simulink model "sim_model"  (R2015b)
settings: Solver=FixedStepDiscrete  SolverMode=SingleTasking  StartTime=0.0  StopTime=sim_len  FixedStep=1  RelTol=1e-3
undefined symbols (not defined in the file): A, B, C, ir_matrix, modulator_reg_1_address, modulator_reg_1_default, modulator_reg_1_num_bits, N_sub
libraries: xbsIndex_r4 x3875
(part 2 of 193)

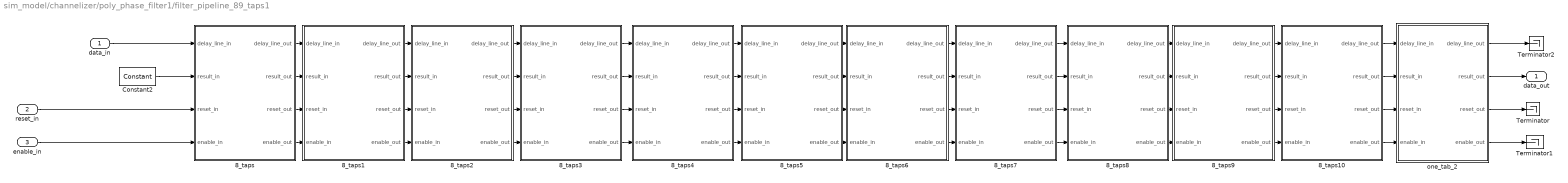
== system sim_model/channelizer/poly_phase_filter1/filter_pipeline_89_taps1 ==
  data_in : Inport
  reset_in : Inport  Port=2
  enable_in : Inport  Port=3
  8_taps : Subsystem  mask{impulse_response_matrix=impulse_response_matrix(0*8+(1:8),:), N_sub=N_sub}
      mask prompts: impulse_response_matrix "Impulse Response Matrix (N_sub x 8)"
  8_taps1 : Subsystem  mask{impulse_response_matrix=impulse_response_matrix(1*8+(1:8),:), N_sub=N_sub}
      mask prompts: impulse_response_matrix "Impulse Response Matrix (N_sub x 8)"
  8_taps10 : Subsystem  mask{impulse_response_matrix=impulse_response_matrix(10*8+(1:8),:), N_sub=N_sub}
      mask prompts: impulse_response_matrix "Impulse Response Matrix (N_sub x 8)"
  8_taps2 : Subsystem  mask{impulse_response_matrix=impulse_response_matrix(2*8+(1:8),:), N_sub=N_sub}
      mask prompts: impulse_response_matrix "Impulse Response Matrix (N_sub x 8)"
  8_taps3 : Subsystem  mask{impulse_response_matrix=impulse_response_matrix(3*8+(1:8),:), N_sub=N_sub}
      mask prompts: impulse_response_matrix "Impulse Response Matrix (N_sub x 8)"
  8_taps4 : Subsystem  mask{impulse_response_matrix=impulse_response_matrix(4*8+(1:8),:), N_sub=N_sub}
      mask prompts: impulse_response_matrix "Impulse Response Matrix (N_sub x 8)"
  8_taps5 : Subsystem  mask{impulse_response_matrix=impulse_response_matrix(5*8+(1:8),:), N_sub=N_sub}
      mask prompts: impulse_response_matrix "Impulse Response Matrix (N_sub x 8)"
  8_taps6 : Subsystem  mask{impulse_response_matrix=impulse_response_matrix(6*8+(1:8),:), N_sub=N_sub}
      mask prompts: impulse_response_matrix "Impulse Response Matrix (N_sub x 8)"
  8_taps7 : Subsystem  mask{impulse_response_matrix=impulse_response_matrix(7*8+(1:8),:), N_sub=N_sub}
      mask prompts: impulse_response_matrix "Impulse Response Matrix (N_sub x 8)"
  8_taps8 : Subsystem  mask{impulse_response_matrix=impulse_response_matrix(8*8+(1:8),:), N_sub=N_sub}
      mask prompts: impulse_response_matrix "Impulse Response Matrix (N_sub x 8)"
  8_taps9 : Subsystem  mask{impulse_response_matrix=impulse_response_matrix(9*8+(1:8),:), N_sub=N_sub}
      mask prompts: impulse_response_matrix "Impulse Response Matrix (N_sub x 8)"
  Constant2 : xbsIndex_r4/Constant  const=0  gui_display_data_type=Fixed-point  arith_type=Signed (2's comp)  n_bits=32  bin_pt=0  preci_type=Single  exp_width=8  frac_width=24  explicit_period=on  period=1  equ=P=C  opselect=C  inp2=PCIN>>17  opr=+  inp1=P  carry=CIN  dbl_ovrd=off  block_type=constant
  Terminator : Terminator
  Terminator1 : Terminator
  Terminator2 : Terminator
  one_tab_2 : Subsystem  mask{impulse_response_matrix=impulse_response_matrix(89,:), N_sub=N_sub}
      mask prompts: impulse_response_matrix "Tab IR"
  data_out : Outport
  wires:
  data_in/1 -> 8_taps/1(delay_line_in)
  reset_in/1 -> 8_taps/3(reset_in)
  enable_in/1 -> 8_taps/4(enable_in)
  Constant2/1 -> 8_taps/2(result_in)
  one_tab_2/4(enable_out) -> Terminator1/1
  one_tab_2/1(delay_line_out) -> Terminator2/1
  one_tab_2/2(result_out) -> data_out/1
  one_tab_2/3(reset_out) -> Terminator/1
  8_taps/1(delay_line_out) -> 8_taps1/1(delay_line_in)
  8_taps/2(result_out) -> 8_taps1/2(result_in)
  8_taps/3(reset_out) -> 8_taps1/3(reset_in)
  8_taps/4(enable_out) -> 8_taps1/4(enable_in)
  8_taps10/1(delay_line_out) -> one_tab_2/1(delay_line_in)
  8_taps10/2(result_out) -> one_tab_2/2(result_in)
  8_taps2/3(reset_out) -> 8_taps3/3(reset_in)
  8_taps2/4(enable_out) -> 8_taps3/4(enable_in)
  8_taps1/1(delay_line_out) -> 8_taps2/1(delay_line_in)
  8_taps1/2(result_out) -> 8_taps2/2(result_in)
  8_taps1/3(reset_out) -> 8_taps2/3(reset_in)
  8_taps1/4(enable_out) -> 8_taps2/4(enable_in)
  8_taps4/2(result_out) -> 8_taps5/2(result_in)
  8_taps4/3(reset_out) -> 8_taps5/3(reset_in)
  8_taps4/4(enable_out) -> 8_taps5/4(enable_in)
  8_taps6/3(reset_out) -> 8_taps7/3(reset_in)
  8_taps6/4(enable_out) -> 8_taps7/4(enable_in)
  8_taps5/2(result_out) -> 8_taps6/2(result_in)
  8_taps5/3(reset_out) -> 8_taps6/3(reset_in)
  8_taps5/4(enable_out) -> 8_taps6/4(enable_in)
  8_taps3/1(delay_line_out) -> 8_taps4/1(delay_line_in)
  8_taps3/2(result_out) -> 8_taps4/2(result_in)
  8_taps3/3(reset_out) -> 8_taps4/3(reset_in)
  8_taps3/4(enable_out) -> 8_taps4/4(enable_in)
  8_taps8/2(result_out) -> 8_taps9/2(result_in)
  8_taps8/3(reset_out) -> 8_taps9/3(reset_in)
  8_taps8/4(enable_out) -> 8_taps9/4(enable_in)
  8_taps9/2(result_out) -> 8_taps10/2(result_in)
  8_taps9/3(reset_out) -> 8_taps10/3(reset_in)
  8_taps9/4(enable_out) -> 8_taps10/4(enable_in)
  8_taps7/1(delay_line_out) -> 8_taps8/1(delay_line_in)
  8_taps7/2(result_out) -> 8_taps8/2(result_in)
  8_taps7/3(reset_out) -> 8_taps8/3(reset_in)
  8_taps7/4(enable_out) -> 8_taps8/4(enable_in)
  8_taps9/1(delay_line_out) -> 8_taps10/1(delay_line_in)
  8_taps10/3(reset_out) -> one_tab_2/3(reset_in)
  8_taps10/4(enable_out) -> one_tab_2/4(enable_in)
  8_taps8/1(delay_line_out) -> 8_taps9/1(delay_line_in)
  8_taps6/1(delay_line_out) -> 8_taps7/1(delay_line_in)
  8_taps6/2(result_out) -> 8_taps7/2(result_in)
  8_taps5/1(delay_line_out) -> 8_taps6/1(delay_line_in)
  8_taps4/1(delay_line_out) -> 8_taps5/1(delay_line_in)
  8_taps2/1(delay_line_out) -> 8_taps3/1(delay_line_in)
  8_taps2/2(result_out) -> 8_taps3/2(result_in)

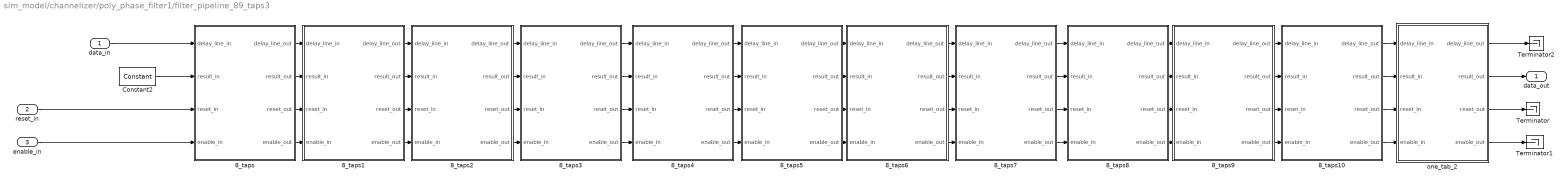
== system sim_model/channelizer/poly_phase_filter1/filter_pipeline_89_taps3 ==
  data_in : Inport
  reset_in : Inport  Port=2
  enable_in : Inport  Port=3
  8_taps : Subsystem  mask{impulse_response_matrix=impulse_response_matrix(0*8+(1:8),:), N_sub=N_sub}
      mask prompts: impulse_response_matrix "Impulse Response Matrix (N_sub x 8)"
  8_taps1 : Subsystem  mask{impulse_response_matrix=impulse_response_matrix(1*8+(1:8),:), N_sub=N_sub}
      mask prompts: impulse_response_matrix "Impulse Response Matrix (N_sub x 8)"
  8_taps10 : Subsystem  mask{impulse_response_matrix=impulse_response_matrix(10*8+(1:8),:), N_sub=N_sub}
      mask prompts: impulse_response_matrix "Impulse Response Matrix (N_sub x 8)"
  8_taps2 : Subsystem  mask{impulse_response_matrix=impulse_response_matrix(2*8+(1:8),:), N_sub=N_sub}
      mask prompts: impulse_response_matrix "Impulse Response Matrix (N_sub x 8)"
  8_taps3 : Subsystem  mask{impulse_response_matrix=impulse_response_matrix(3*8+(1:8),:), N_sub=N_sub}
      mask prompts: impulse_response_matrix "Impulse Response Matrix (N_sub x 8)"
  8_taps4 : Subsystem  mask{impulse_response_matrix=impulse_response_matrix(4*8+(1:8),:), N_sub=N_sub}
      mask prompts: impulse_response_matrix "Impulse Response Matrix (N_sub x 8)"
  8_taps5 : Subsystem  mask{impulse_response_matrix=impulse_response_matrix(5*8+(1:8),:), N_sub=N_sub}
      mask prompts: impulse_response_matrix "Impulse Response Matrix (N_sub x 8)"
  8_taps6 : Subsystem  mask{impulse_response_matrix=impulse_response_matrix(6*8+(1:8),:), N_sub=N_sub}
      mask prompts: impulse_response_matrix "Impulse Response Matrix (N_sub x 8)"
  8_taps7 : Subsystem  mask{impulse_response_matrix=impulse_response_matrix(7*8+(1:8),:), N_sub=N_sub}
      mask prompts: impulse_response_matrix "Impulse Response Matrix (N_sub x 8)"
  8_taps8 : Subsystem  mask{impulse_response_matrix=impulse_response_matrix(8*8+(1:8),:), N_sub=N_sub}
      mask prompts: impulse_response_matrix "Impulse Response Matrix (N_sub x 8)"
  8_taps9 : Subsystem  mask{impulse_response_matrix=impulse_response_matrix(9*8+(1:8),:), N_sub=N_sub}
      mask prompts: impulse_response_matrix "Impulse Response Matrix (N_sub x 8)"
  Constant2 : xbsIndex_r4/Constant  const=0  gui_display_data_type=Fixed-point  arith_type=Signed (2's comp)  n_bits=32  bin_pt=0  preci_type=Single  exp_width=8  frac_width=24  explicit_period=on  period=1  equ=P=C  opselect=C  inp2=PCIN>>17  opr=+  inp1=P  carry=CIN  dbl_ovrd=off  block_type=constant
  Terminator : Terminator
  Terminator1 : Terminator
  Terminator2 : Terminator
  one_tab_2 : Subsystem  mask{impulse_response_matrix=impulse_response_matrix(89,:), N_sub=N_sub}
      mask prompts: impulse_response_matrix "Tab IR"
  data_out : Outport
  wires:
  data_in/1 -> 8_taps/1(delay_line_in)
  reset_in/1 -> 8_taps/3(reset_in)
  enable_in/1 -> 8_taps/4(enable_in)
  Constant2/1 -> 8_taps/2(result_in)
  one_tab_2/4(enable_out) -> Terminator1/1
  one_tab_2/1(delay_line_out) -> Terminator2/1
  one_tab_2/2(result_out) -> data_out/1
  one_tab_2/3(reset_out) -> Terminator/1
  8_taps/1(delay_line_out) -> 8_taps1/1(delay_line_in)
  8_taps/2(result_out) -> 8_taps1/2(result_in)
  8_taps/3(reset_out) -> 8_taps1/3(reset_in)
  8_taps/4(enable_out) -> 8_taps1/4(enable_in)
  8_taps10/1(delay_line_out) -> one_tab_2/1(delay_line_in)
  8_taps10/2(result_out) -> one_tab_2/2(result_in)
  8_taps2/3(reset_out) -> 8_taps3/3(reset_in)
  8_taps2/4(enable_out) -> 8_taps3/4(enable_in)
  8_taps1/1(delay_line_out) -> 8_taps2/1(delay_line_in)
  8_taps1/2(result_out) -> 8_taps2/2(result_in)
  8_taps1/3(reset_out) -> 8_taps2/3(reset_in)
  8_taps1/4(enable_out) -> 8_taps2/4(enable_in)
  8_taps4/2(result_out) -> 8_taps5/2(result_in)
  8_taps4/3(reset_out) -> 8_taps5/3(reset_in)
  8_taps4/4(enable_out) -> 8_taps5/4(enable_in)
  8_taps6/3(reset_out) -> 8_taps7/3(reset_in)
  8_taps6/4(enable_out) -> 8_taps7/4(enable_in)
  8_taps5/2(result_out) -> 8_taps6/2(result_in)
  8_taps5/3(reset_out) -> 8_taps6/3(reset_in)
  8_taps5/4(enable_out) -> 8_taps6/4(enable_in)
  8_taps3/1(delay_line_out) -> 8_taps4/1(delay_line_in)
  8_taps3/2(result_out) -> 8_taps4/2(result_in)
  8_taps3/3(reset_out) -> 8_taps4/3(reset_in)
  8_taps3/4(enable_out) -> 8_taps4/4(enable_in)
  8_taps8/2(result_out) -> 8_taps9/2(result_in)
  8_taps8/3(reset_out) -> 8_taps9/3(reset_in)
  8_taps8/4(enable_out) -> 8_taps9/4(enable_in)
  8_taps9/2(result_out) -> 8_taps10/2(result_in)
  8_taps9/3(reset_out) -> 8_taps10/3(reset_in)
  8_taps9/4(enable_out) -> 8_taps10/4(enable_in)
  8_taps7/1(delay_line_out) -> 8_taps8/1(delay_line_in)
  8_taps7/2(result_out) -> 8_taps8/2(result_in)
  8_taps7/3(reset_out) -> 8_taps8/3(reset_in)
  8_taps7/4(enable_out) -> 8_taps8/4(enable_in)
  8_taps9/1(delay_line_out) -> 8_taps10/1(delay_line_in)
  8_taps10/3(reset_out) -> one_tab_2/3(reset_in)
  8_taps10/4(enable_out) -> one_tab_2/4(enable_in)
  8_taps8/1(delay_line_out) -> 8_taps9/1(delay_line_in)
  8_taps6/1(delay_line_out) -> 8_taps7/1(delay_line_in)
  8_taps6/2(result_out) -> 8_taps7/2(result_in)
  8_taps5/1(delay_line_out) -> 8_taps6/1(delay_line_in)
  8_taps4/1(delay_line_out) -> 8_taps5/1(delay_line_in)
  8_taps2/1(delay_line_out) -> 8_taps3/1(delay_line_in)
  8_taps2/2(result_out) -> 8_taps3/2(result_in)

== system sim_model/channelizer/poly_phase_filter1/filter_pipeline_89_taps1/8_taps ==
  delay_line_in : Inport
  result_in : Inport  Port=2
  reset_in : Inport  Port=3
  enable_in : Inport  Port=4
  one_tab_1 : Subsystem  mask{impulse_response_matrix=impulse_response_matrix(2,:), N_sub=N_sub}
      mask prompts: impulse_response_matrix "Tab IR"
  one_tab_2 : Subsystem  mask{impulse_response_matrix=impulse_response_matrix(4,:), N_sub=N_sub}
      mask prompts: impulse_response_matrix "Tab IR"
  one_tab_3 : Subsystem  mask{impulse_response_matrix=impulse_response_matrix(3,:), N_sub=N_sub}
      mask prompts: impulse_response_matrix "Tab IR"
  one_tab_4 : Subsystem  mask{impulse_response_matrix=impulse_response_matrix(6,:), N_sub=N_sub}
      mask prompts: impulse_response_matrix "Tab IR"
  one_tab_5 : Subsystem  mask{impulse_response_matrix=impulse_response_matrix(5,:), N_sub=N_sub}
      mask prompts: impulse_response_matrix "Tab IR"
  one_tab_6 : Subsystem  mask{impulse_response_matrix=impulse_response_matrix(8,:), N_sub=N_sub}
      mask prompts: impulse_response_matrix "Tab IR"
  one_tab_7 : Subsystem  mask{impulse_response_matrix=impulse_response_matrix(7,:), N_sub=N_sub}
      mask prompts: impulse_response_matrix "Tab IR"
  one_tab_8 : Subsystem  mask{impulse_response_matrix=impulse_response_matrix(1,:), N_sub=N_sub}
      mask prompts: impulse_response_matrix "Tab IR"
  delay_line_out : Outport
  result_out : Outport  Port=2
  reset_out : Outport  Port=3
  enable_out : Outport  Port=4
  wires:
  one_tab_6/1(delay_line_out) -> delay_line_out/1
  one_tab_6/2(result_out) -> result_out/1
  one_tab_6/3(reset_out) -> reset_out/1
  result_in/1 -> one_tab_8/2(result_in)
  delay_line_in/1 -> one_tab_8/1(delay_line_in)
  reset_in/1 -> one_tab_8/3(reset_in)
  enable_in/1 -> one_tab_8/4(enable_in)
  one_tab_6/4(enable_out) -> enable_out/1
  one_tab_8/1(delay_line_out) -> one_tab_1/1(delay_line_in)
  one_tab_8/2(result_out) -> one_tab_1/2(result_in)
  one_tab_8/3(reset_out) -> one_tab_1/3(reset_in)
  one_tab_8/4(enable_out) -> one_tab_1/4(enable_in)
  one_tab_3/1(delay_line_out) -> one_tab_2/1(delay_line_in)
  one_tab_3/2(result_out) -> one_tab_2/2(result_in)
  one_tab_3/3(reset_out) -> one_tab_2/3(reset_in)
  one_tab_3/4(enable_out) -> one_tab_2/4(enable_in)
  one_tab_1/1(delay_line_out) -> one_tab_3/1(delay_line_in)
  one_tab_1/2(result_out) -> one_tab_3/2(result_in)
  one_tab_1/3(reset_out) -> one_tab_3/3(reset_in)
  one_tab_1/4(enable_out) -> one_tab_3/4(enable_in)
  one_tab_5/1(delay_line_out) -> one_tab_4/1(delay_line_in)
  one_tab_5/2(result_out) -> one_tab_4/2(result_in)
  one_tab_5/3(reset_out) -> one_tab_4/3(reset_in)
  one_tab_5/4(enable_out) -> one_tab_4/4(enable_in)
  one_tab_2/1(delay_line_out) -> one_tab_5/1(delay_line_in)
  one_tab_2/2(result_out) -> one_tab_5/2(result_in)
  one_tab_2/3(reset_out) -> one_tab_5/3(reset_in)
  one_tab_2/4(enable_out) -> one_tab_5/4(enable_in)
  one_tab_7/1(delay_line_out) -> one_tab_6/1(delay_line_in)
  one_tab_7/2(result_out) -> one_tab_6/2(result_in)
  one_tab_7/3(reset_out) -> one_tab_6/3(reset_in)
  one_tab_7/4(enable_out) -> one_tab_6/4(enable_in)
  one_tab_4/1(delay_line_out) -> one_tab_7/1(delay_line_in)
  one_tab_4/2(result_out) -> one_tab_7/2(result_in)
  one_tab_4/3(reset_out) -> one_tab_7/3(reset_in)
  one_tab_4/4(enable_out) -> one_tab_7/4(enable_in)

== system sim_model/channelizer/poly_phase_filter1/filter_pipeline_89_taps1/8_taps1 ==
  delay_line_in : Inport
  result_in : Inport  Port=2
  reset_in : Inport  Port=3
  enable_in : Inport  Port=4
  one_tab_1 : Subsystem  mask{impulse_response_matrix=impulse_response_matrix(2,:), N_sub=N_sub}
      mask prompts: impulse_response_matrix "Tab IR"
  one_tab_2 : Subsystem  mask{impulse_response_matrix=impulse_response_matrix(4,:), N_sub=N_sub}
      mask prompts: impulse_response_matrix "Tab IR"
  one_tab_3 : Subsystem  mask{impulse_response_matrix=impulse_response_matrix(3,:), N_sub=N_sub}
      mask prompts: impulse_response_matrix "Tab IR"
  one_tab_4 : Subsystem  mask{impulse_response_matrix=impulse_response_matrix(6,:), N_sub=N_sub}
      mask prompts: impulse_response_matrix "Tab IR"
  one_tab_5 : Subsystem  mask{impulse_response_matrix=impulse_response_matrix(5,:), N_sub=N_sub}
      mask prompts: impulse_response_matrix "Tab IR"
  one_tab_6 : Subsystem  mask{impulse_response_matrix=impulse_response_matrix(8,:), N_sub=N_sub}
      mask prompts: impulse_response_matrix "Tab IR"
  one_tab_7 : Subsystem  mask{impulse_response_matrix=impulse_response_matrix(7,:), N_sub=N_sub}
      mask prompts: impulse_response_matrix "Tab IR"
  one_tab_8 : Subsystem  mask{impulse_response_matrix=impulse_response_matrix(1,:), N_sub=N_sub}
      mask prompts: impulse_response_matrix "Tab IR"
  delay_line_out : Outport
  result_out : Outport  Port=2
  reset_out : Outport  Port=3
  enable_out : Outport  Port=4
  wires:
  one_tab_6/1(delay_line_out) -> delay_line_out/1
  one_tab_6/2(result_out) -> result_out/1
  one_tab_6/3(reset_out) -> reset_out/1
  result_in/1 -> one_tab_8/2(result_in)
  delay_line_in/1 -> one_tab_8/1(delay_line_in)
  reset_in/1 -> one_tab_8/3(reset_in)
  enable_in/1 -> one_tab_8/4(enable_in)
  one_tab_6/4(enable_out) -> enable_out/1
  one_tab_8/1(delay_line_out) -> one_tab_1/1(delay_line_in)
  one_tab_8/2(result_out) -> one_tab_1/2(result_in)
  one_tab_8/3(reset_out) -> one_tab_1/3(reset_in)
  one_tab_8/4(enable_out) -> one_tab_1/4(enable_in)
  one_tab_3/1(delay_line_out) -> one_tab_2/1(delay_line_in)
  one_tab_3/2(result_out) -> one_tab_2/2(result_in)
  one_tab_3/3(reset_out) -> one_tab_2/3(reset_in)
  one_tab_3/4(enable_out) -> one_tab_2/4(enable_in)
  one_tab_1/1(delay_line_out) -> one_tab_3/1(delay_line_in)
  one_tab_1/2(result_out) -> one_tab_3/2(result_in)
  one_tab_1/3(reset_out) -> one_tab_3/3(reset_in)
  one_tab_1/4(enable_out) -> one_tab_3/4(enable_in)
  one_tab_5/1(delay_line_out) -> one_tab_4/1(delay_line_in)
  one_tab_5/2(result_out) -> one_tab_4/2(result_in)
  one_tab_5/3(reset_out) -> one_tab_4/3(reset_in)
  one_tab_5/4(enable_out) -> one_tab_4/4(enable_in)
  one_tab_2/1(delay_line_out) -> one_tab_5/1(delay_line_in)
  one_tab_2/2(result_out) -> one_tab_5/2(result_in)
  one_tab_2/3(reset_out) -> one_tab_5/3(reset_in)
  one_tab_2/4(enable_out) -> one_tab_5/4(enable_in)
  one_tab_7/1(delay_line_out) -> one_tab_6/1(delay_line_in)
  one_tab_7/2(result_out) -> one_tab_6/2(result_in)
  one_tab_7/3(reset_out) -> one_tab_6/3(reset_in)
  one_tab_7/4(enable_out) -> one_tab_6/4(enable_in)
  one_tab_4/1(delay_line_out) -> one_tab_7/1(delay_line_in)
  one_tab_4/2(result_out) -> one_tab_7/2(result_in)
  one_tab_4/3(reset_out) -> one_tab_7/3(reset_in)
  one_tab_4/4(enable_out) -> one_tab_7/4(enable_in)

== system sim_model/channelizer/poly_phase_filter1/filter_pipeline_89_taps1/8_taps10 ==
  delay_line_in : Inport
  result_in : Inport  Port=2
  reset_in : Inport  Port=3
  enable_in : Inport  Port=4
  one_tab_1 : Subsystem  mask{impulse_response_matrix=impulse_response_matrix(2,:), N_sub=N_sub}
      mask prompts: impulse_response_matrix "Tab IR"
  one_tab_2 : Subsystem  mask{impulse_response_matrix=impulse_response_matrix(4,:), N_sub=N_sub}
      mask prompts: impulse_response_matrix "Tab IR"
  one_tab_3 : Subsystem  mask{impulse_response_matrix=impulse_response_matrix(3,:), N_sub=N_sub}
      mask prompts: impulse_response_matrix "Tab IR"
  one_tab_4 : Subsystem  mask{impulse_response_matrix=impulse_response_matrix(6,:), N_sub=N_sub}
      mask prompts: impulse_response_matrix "Tab IR"
  one_tab_5 : Subsystem  mask{impulse_response_matrix=impulse_response_matrix(5,:), N_sub=N_sub}
      mask prompts: impulse_response_matrix "Tab IR"
  one_tab_6 : Subsystem  mask{impulse_response_matrix=impulse_response_matrix(8,:), N_sub=N_sub}
      mask prompts: impulse_response_matrix "Tab IR"
  one_tab_7 : Subsystem  mask{impulse_response_matrix=impulse_response_matrix(7,:), N_sub=N_sub}
      mask prompts: impulse_response_matrix "Tab IR"
  one_tab_8 : Subsystem  mask{impulse_response_matrix=impulse_response_matrix(1,:), N_sub=N_sub}
      mask prompts: impulse_response_matrix "Tab IR"
  delay_line_out : Outport
  result_out : Outport  Port=2
  reset_out : Outport  Port=3
  enable_out : Outport  Port=4
  wires:
  one_tab_6/1(delay_line_out) -> delay_line_out/1
  one_tab_6/2(result_out) -> result_out/1
  one_tab_6/3(reset_out) -> reset_out/1
  result_in/1 -> one_tab_8/2(result_in)
  delay_line_in/1 -> one_tab_8/1(delay_line_in)
  reset_in/1 -> one_tab_8/3(reset_in)
  enable_in/1 -> one_tab_8/4(enable_in)
  one_tab_6/4(enable_out) -> enable_out/1
  one_tab_8/1(delay_line_out) -> one_tab_1/1(delay_line_in)
  one_tab_8/2(result_out) -> one_tab_1/2(result_in)
  one_tab_8/3(reset_out) -> one_tab_1/3(reset_in)
  one_tab_8/4(enable_out) -> one_tab_1/4(enable_in)
  one_tab_3/1(delay_line_out) -> one_tab_2/1(delay_line_in)
  one_tab_3/2(result_out) -> one_tab_2/2(result_in)
  one_tab_3/3(reset_out) -> one_tab_2/3(reset_in)
  one_tab_3/4(enable_out) -> one_tab_2/4(enable_in)
  one_tab_1/1(delay_line_out) -> one_tab_3/1(delay_line_in)
  one_tab_1/2(result_out) -> one_tab_3/2(result_in)
  one_tab_1/3(reset_out) -> one_tab_3/3(reset_in)
  one_tab_1/4(enable_out) -> one_tab_3/4(enable_in)
  one_tab_5/1(delay_line_out) -> one_tab_4/1(delay_line_in)
  one_tab_5/2(result_out) -> one_tab_4/2(result_in)
  one_tab_5/3(reset_out) -> one_tab_4/3(reset_in)
  one_tab_5/4(enable_out) -> one_tab_4/4(enable_in)
  one_tab_2/1(delay_line_out) -> one_tab_5/1(delay_line_in)
  one_tab_2/2(result_out) -> one_tab_5/2(result_in)
  one_tab_2/3(reset_out) -> one_tab_5/3(reset_in)
  one_tab_2/4(enable_out) -> one_tab_5/4(enable_in)
  one_tab_7/1(delay_line_out) -> one_tab_6/1(delay_line_in)
  one_tab_7/2(result_out) -> one_tab_6/2(result_in)
  one_tab_7/3(reset_out) -> one_tab_6/3(reset_in)
  one_tab_7/4(enable_out) -> one_tab_6/4(enable_in)
  one_tab_4/1(delay_line_out) -> one_tab_7/1(delay_line_in)
  one_tab_4/2(result_out) -> one_tab_7/2(result_in)
  one_tab_4/3(reset_out) -> one_tab_7/3(reset_in)
  one_tab_4/4(enable_out) -> one_tab_7/4(enable_in)

== system sim_model/channelizer/poly_phase_filter1/filter_pipeline_89_taps1/8_taps2 ==
  delay_line_in : Inport
  result_in : Inport  Port=2
  reset_in : Inport  Port=3
  enable_in : Inport  Port=4
  one_tab_1 : Subsystem  mask{impulse_response_matrix=impulse_response_matrix(2,:), N_sub=N_sub}
      mask prompts: impulse_response_matrix "Tab IR"
  one_tab_2 : Subsystem  mask{impulse_response_matrix=impulse_response_matrix(4,:), N_sub=N_sub}
      mask prompts: impulse_response_matrix "Tab IR"
  one_tab_3 : Subsystem  mask{impulse_response_matrix=impulse_response_matrix(3,:), N_sub=N_sub}
      mask prompts: impulse_response_matrix "Tab IR"
  one_tab_4 : Subsystem  mask{impulse_response_matrix=impulse_response_matrix(6,:), N_sub=N_sub}
      mask prompts: impulse_response_matrix "Tab IR"
  one_tab_5 : Subsystem  mask{impulse_response_matrix=impulse_response_matrix(5,:), N_sub=N_sub}
      mask prompts: impulse_response_matrix "Tab IR"
  one_tab_6 : Subsystem  mask{impulse_response_matrix=impulse_response_matrix(8,:), N_sub=N_sub}
      mask prompts: impulse_response_matrix "Tab IR"
  one_tab_7 : Subsystem  mask{impulse_response_matrix=impulse_response_matrix(7,:), N_sub=N_sub}
      mask prompts: impulse_response_matrix "Tab IR"
  one_tab_8 : Subsystem  mask{impulse_response_matrix=impulse_response_matrix(1,:), N_sub=N_sub}
      mask prompts: impulse_response_matrix "Tab IR"
  delay_line_out : Outport
  result_out : Outport  Port=2
  reset_out : Outport  Port=3
  enable_out : Outport  Port=4
  wires:
  one_tab_6/1(delay_line_out) -> delay_line_out/1
  one_tab_6/2(result_out) -> result_out/1
  one_tab_6/3(reset_out) -> reset_out/1
  result_in/1 -> one_tab_8/2(result_in)
  delay_line_in/1 -> one_tab_8/1(delay_line_in)
  reset_in/1 -> one_tab_8/3(reset_in)
  enable_in/1 -> one_tab_8/4(enable_in)
  one_tab_6/4(enable_out) -> enable_out/1
  one_tab_8/1(delay_line_out) -> one_tab_1/1(delay_line_in)
  one_tab_8/2(result_out) -> one_tab_1/2(result_in)
  one_tab_8/3(reset_out) -> one_tab_1/3(reset_in)
  one_tab_8/4(enable_out) -> one_tab_1/4(enable_in)
  one_tab_3/1(delay_line_out) -> one_tab_2/1(delay_line_in)
  one_tab_3/2(result_out) -> one_tab_2/2(result_in)
  one_tab_3/3(reset_out) -> one_tab_2/3(reset_in)
  one_tab_3/4(enable_out) -> one_tab_2/4(enable_in)
  one_tab_1/1(delay_line_out) -> one_tab_3/1(delay_line_in)
  one_tab_1/2(result_out) -> one_tab_3/2(result_in)
  one_tab_1/3(reset_out) -> one_tab_3/3(reset_in)
  one_tab_1/4(enable_out) -> one_tab_3/4(enable_in)
  one_tab_5/1(delay_line_out) -> one_tab_4/1(delay_line_in)
  one_tab_5/2(result_out) -> one_tab_4/2(result_in)
  one_tab_5/3(reset_out) -> one_tab_4/3(reset_in)
  one_tab_5/4(enable_out) -> one_tab_4/4(enable_in)
  one_tab_2/1(delay_line_out) -> one_tab_5/1(delay_line_in)
  one_tab_2/2(result_out) -> one_tab_5/2(result_in)
  one_tab_2/3(reset_out) -> one_tab_5/3(reset_in)
  one_tab_2/4(enable_out) -> one_tab_5/4(enable_in)
  one_tab_7/1(delay_line_out) -> one_tab_6/1(delay_line_in)
  one_tab_7/2(result_out) -> one_tab_6/2(result_in)
  one_tab_7/3(reset_out) -> one_tab_6/3(reset_in)
  one_tab_7/4(enable_out) -> one_tab_6/4(enable_in)
  one_tab_4/1(delay_line_out) -> one_tab_7/1(delay_line_in)
  one_tab_4/2(result_out) -> one_tab_7/2(result_in)
  one_tab_4/3(reset_out) -> one_tab_7/3(reset_in)
  one_tab_4/4(enable_out) -> one_tab_7/4(enable_in)

== system sim_model/channelizer/poly_phase_filter1/filter_pipeline_89_taps1/8_taps3 ==
  delay_line_in : Inport
  result_in : Inport  Port=2
  reset_in : Inport  Port=3
  enable_in : Inport  Port=4
  one_tab_1 : Subsystem  mask{impulse_response_matrix=impulse_response_matrix(2,:), N_sub=N_sub}
      mask prompts: impulse_response_matrix "Tab IR"
  one_tab_2 : Subsystem  mask{impulse_response_matrix=impulse_response_matrix(4,:), N_sub=N_sub}
      mask prompts: impulse_response_matrix "Tab IR"
  one_tab_3 : Subsystem  mask{impulse_response_matrix=impulse_response_matrix(3,:), N_sub=N_sub}
      mask prompts: impulse_response_matrix "Tab IR"
  one_tab_4 : Subsystem  mask{impulse_response_matrix=impulse_response_matrix(6,:), N_sub=N_sub}
      mask prompts: impulse_response_matrix "Tab IR"
  one_tab_5 : Subsystem  mask{impulse_response_matrix=impulse_response_matrix(5,:), N_sub=N_sub}
      mask prompts: impulse_response_matrix "Tab IR"
  one_tab_6 : Subsystem  mask{impulse_response_matrix=impulse_response_matrix(8,:), N_sub=N_sub}
      mask prompts: impulse_response_matrix "Tab IR"
  one_tab_7 : Subsystem  mask{impulse_response_matrix=impulse_response_matrix(7,:), N_sub=N_sub}
      mask prompts: impulse_response_matrix "Tab IR"
  one_tab_8 : Subsystem  mask{impulse_response_matrix=impulse_response_matrix(1,:), N_sub=N_sub}
      mask prompts: impulse_response_matrix "Tab IR"
  delay_line_out : Outport
  result_out : Outport  Port=2
  reset_out : Outport  Port=3
  enable_out : Outport  Port=4
  wires:
  one_tab_6/1(delay_line_out) -> delay_line_out/1
  one_tab_6/2(result_out) -> result_out/1
  one_tab_6/3(reset_out) -> reset_out/1
  result_in/1 -> one_tab_8/2(result_in)
  delay_line_in/1 -> one_tab_8/1(delay_line_in)
  reset_in/1 -> one_tab_8/3(reset_in)
  enable_in/1 -> one_tab_8/4(enable_in)
  one_tab_6/4(enable_out) -> enable_out/1
  one_tab_8/1(delay_line_out) -> one_tab_1/1(delay_line_in)
  one_tab_8/2(result_out) -> one_tab_1/2(result_in)
  one_tab_8/3(reset_out) -> one_tab_1/3(reset_in)
  one_tab_8/4(enable_out) -> one_tab_1/4(enable_in)
  one_tab_3/1(delay_line_out) -> one_tab_2/1(delay_line_in)
  one_tab_3/2(result_out) -> one_tab_2/2(result_in)
  one_tab_3/3(reset_out) -> one_tab_2/3(reset_in)
  one_tab_3/4(enable_out) -> one_tab_2/4(enable_in)
  one_tab_1/1(delay_line_out) -> one_tab_3/1(delay_line_in)
  one_tab_1/2(result_out) -> one_tab_3/2(result_in)
  one_tab_1/3(reset_out) -> one_tab_3/3(reset_in)
  one_tab_1/4(enable_out) -> one_tab_3/4(enable_in)
  one_tab_5/1(delay_line_out) -> one_tab_4/1(delay_line_in)
  one_tab_5/2(result_out) -> one_tab_4/2(result_in)
  one_tab_5/3(reset_out) -> one_tab_4/3(reset_in)
  one_tab_5/4(enable_out) -> one_tab_4/4(enable_in)
  one_tab_2/1(delay_line_out) -> one_tab_5/1(delay_line_in)
  one_tab_2/2(result_out) -> one_tab_5/2(result_in)
  one_tab_2/3(reset_out) -> one_tab_5/3(reset_in)
  one_tab_2/4(enable_out) -> one_tab_5/4(enable_in)
  one_tab_7/1(delay_line_out) -> one_tab_6/1(delay_line_in)
  one_tab_7/2(result_out) -> one_tab_6/2(result_in)
  one_tab_7/3(reset_out) -> one_tab_6/3(reset_in)
  one_tab_7/4(enable_out) -> one_tab_6/4(enable_in)
  one_tab_4/1(delay_line_out) -> one_tab_7/1(delay_line_in)
  one_tab_4/2(result_out) -> one_tab_7/2(result_in)
  one_tab_4/3(reset_out) -> one_tab_7/3(reset_in)
  one_tab_4/4(enable_out) -> one_tab_7/4(enable_in)

== system sim_model/channelizer/poly_phase_filter1/filter_pipeline_89_taps1/8_taps4 ==
  delay_line_in : Inport
  result_in : Inport  Port=2
  reset_in : Inport  Port=3
  enable_in : Inport  Port=4
  one_tab_1 : Subsystem  mask{impulse_response_matrix=impulse_response_matrix(2,:), N_sub=N_sub}
      mask prompts: impulse_response_matrix "Tab IR"
  one_tab_2 : Subsystem  mask{impulse_response_matrix=impulse_response_matrix(4,:), N_sub=N_sub}
      mask prompts: impulse_response_matrix "Tab IR"
  one_tab_3 : Subsystem  mask{impulse_response_matrix=impulse_response_matrix(3,:), N_sub=N_sub}
      mask prompts: impulse_response_matrix "Tab IR"
  one_tab_4 : Subsystem  mask{impulse_response_matrix=impulse_response_matrix(6,:), N_sub=N_sub}
      mask prompts: impulse_response_matrix "Tab IR"
  one_tab_5 : Subsystem  mask{impulse_response_matrix=impulse_response_matrix(5,:), N_sub=N_sub}
      mask prompts: impulse_response_matrix "Tab IR"
  one_tab_6 : Subsystem  mask{impulse_response_matrix=impulse_response_matrix(8,:), N_sub=N_sub}
      mask prompts: impulse_response_matrix "Tab IR"
  one_tab_7 : Subsystem  mask{impulse_response_matrix=impulse_response_matrix(7,:), N_sub=N_sub}
      mask prompts: impulse_response_matrix "Tab IR"
  one_tab_8 : Subsystem  mask{impulse_response_matrix=impulse_response_matrix(1,:), N_sub=N_sub}
      mask prompts: impulse_response_matrix "Tab IR"
  delay_line_out : Outport
  result_out : Outport  Port=2
  reset_out : Outport  Port=3
  enable_out : Outport  Port=4
  wires:
  one_tab_6/1(delay_line_out) -> delay_line_out/1
  one_tab_6/2(result_out) -> result_out/1
  one_tab_6/3(reset_out) -> reset_out/1
  result_in/1 -> one_tab_8/2(result_in)
  delay_line_in/1 -> one_tab_8/1(delay_line_in)
  reset_in/1 -> one_tab_8/3(reset_in)
  enable_in/1 -> one_tab_8/4(enable_in)
  one_tab_6/4(enable_out) -> enable_out/1
  one_tab_8/1(delay_line_out) -> one_tab_1/1(delay_line_in)
  one_tab_8/2(result_out) -> one_tab_1/2(result_in)
  one_tab_8/3(reset_out) -> one_tab_1/3(reset_in)
  one_tab_8/4(enable_out) -> one_tab_1/4(enable_in)
  one_tab_3/1(delay_line_out) -> one_tab_2/1(delay_line_in)
  one_tab_3/2(result_out) -> one_tab_2/2(result_in)
  one_tab_3/3(reset_out) -> one_tab_2/3(reset_in)
  one_tab_3/4(enable_out) -> one_tab_2/4(enable_in)
  one_tab_1/1(delay_line_out) -> one_tab_3/1(delay_line_in)
  one_tab_1/2(result_out) -> one_tab_3/2(result_in)
  one_tab_1/3(reset_out) -> one_tab_3/3(reset_in)
  one_tab_1/4(enable_out) -> one_tab_3/4(enable_in)
  one_tab_5/1(delay_line_out) -> one_tab_4/1(delay_line_in)
  one_tab_5/2(result_out) -> one_tab_4/2(result_in)
  one_tab_5/3(reset_out) -> one_tab_4/3(reset_in)
  one_tab_5/4(enable_out) -> one_tab_4/4(enable_in)
  one_tab_2/1(delay_line_out) -> one_tab_5/1(delay_line_in)
  one_tab_2/2(result_out) -> one_tab_5/2(result_in)
  one_tab_2/3(reset_out) -> one_tab_5/3(reset_in)
  one_tab_2/4(enable_out) -> one_tab_5/4(enable_in)
  one_tab_7/1(delay_line_out) -> one_tab_6/1(delay_line_in)
  one_tab_7/2(result_out) -> one_tab_6/2(result_in)
  one_tab_7/3(reset_out) -> one_tab_6/3(reset_in)
  one_tab_7/4(enable_out) -> one_tab_6/4(enable_in)
  one_tab_4/1(delay_line_out) -> one_tab_7/1(delay_line_in)
  one_tab_4/2(result_out) -> one_tab_7/2(result_in)
  one_tab_4/3(reset_out) -> one_tab_7/3(reset_in)
  one_tab_4/4(enable_out) -> one_tab_7/4(enable_in)

== system sim_model/channelizer/poly_phase_filter1/filter_pipeline_89_taps1/8_taps5 ==
  delay_line_in : Inport
  result_in : Inport  Port=2
  reset_in : Inport  Port=3
  enable_in : Inport  Port=4
  one_tab_1 : Subsystem  mask{impulse_response_matrix=impulse_response_matrix(2,:), N_sub=N_sub}
      mask prompts: impulse_response_matrix "Tab IR"
  one_tab_2 : Subsystem  mask{impulse_response_matrix=impulse_response_matrix(4,:), N_sub=N_sub}
      mask prompts: impulse_response_matrix "Tab IR"
  one_tab_3 : Subsystem  mask{impulse_response_matrix=impulse_response_matrix(3,:), N_sub=N_sub}
      mask prompts: impulse_response_matrix "Tab IR"
  one_tab_4 : Subsystem  mask{impulse_response_matrix=impulse_response_matrix(6,:), N_sub=N_sub}
      mask prompts: impulse_response_matrix "Tab IR"
  one_tab_5 : Subsystem  mask{impulse_response_matrix=impulse_response_matrix(5,:), N_sub=N_sub}
      mask prompts: impulse_response_matrix "Tab IR"
  one_tab_6 : Subsystem  mask{impulse_response_matrix=impulse_response_matrix(8,:), N_sub=N_sub}
      mask prompts: impulse_response_matrix "Tab IR"
  one_tab_7 : Subsystem  mask{impulse_response_matrix=impulse_response_matrix(7,:), N_sub=N_sub}
      mask prompts: impulse_response_matrix "Tab IR"
  one_tab_8 : Subsystem  mask{impulse_response_matrix=impulse_response_matrix(1,:), N_sub=N_sub}
      mask prompts: impulse_response_matrix "Tab IR"
  delay_line_out : Outport
  result_out : Outport  Port=2
  reset_out : Outport  Port=3
  enable_out : Outport  Port=4
  wires:
  one_tab_6/1(delay_line_out) -> delay_line_out/1
  one_tab_6/2(result_out) -> result_out/1
  one_tab_6/3(reset_out) -> reset_out/1
  result_in/1 -> one_tab_8/2(result_in)
  delay_line_in/1 -> one_tab_8/1(delay_line_in)
  reset_in/1 -> one_tab_8/3(reset_in)
  enable_in/1 -> one_tab_8/4(enable_in)
  one_tab_6/4(enable_out) -> enable_out/1
  one_tab_8/1(delay_line_out) -> one_tab_1/1(delay_line_in)
  one_tab_8/2(result_out) -> one_tab_1/2(result_in)
  one_tab_8/3(reset_out) -> one_tab_1/3(reset_in)
  one_tab_8/4(enable_out) -> one_tab_1/4(enable_in)
  one_tab_3/1(delay_line_out) -> one_tab_2/1(delay_line_in)
  one_tab_3/2(result_out) -> one_tab_2/2(result_in)
  one_tab_3/3(reset_out) -> one_tab_2/3(reset_in)
  one_tab_3/4(enable_out) -> one_tab_2/4(enable_in)
  one_tab_1/1(delay_line_out) -> one_tab_3/1(delay_line_in)
  one_tab_1/2(result_out) -> one_tab_3/2(result_in)
  one_tab_1/3(reset_out) -> one_tab_3/3(reset_in)
  one_tab_1/4(enable_out) -> one_tab_3/4(enable_in)
  one_tab_5/1(delay_line_out) -> one_tab_4/1(delay_line_in)
  one_tab_5/2(result_out) -> one_tab_4/2(result_in)
  one_tab_5/3(reset_out) -> one_tab_4/3(reset_in)
  one_tab_5/4(enable_out) -> one_tab_4/4(enable_in)
  one_tab_2/1(delay_line_out) -> one_tab_5/1(delay_line_in)
  one_tab_2/2(result_out) -> one_tab_5/2(result_in)
  one_tab_2/3(reset_out) -> one_tab_5/3(reset_in)
  one_tab_2/4(enable_out) -> one_tab_5/4(enable_in)
  one_tab_7/1(delay_line_out) -> one_tab_6/1(delay_line_in)
  one_tab_7/2(result_out) -> one_tab_6/2(result_in)
  one_tab_7/3(reset_out) -> one_tab_6/3(reset_in)
  one_tab_7/4(enable_out) -> one_tab_6/4(enable_in)
  one_tab_4/1(delay_line_out) -> one_tab_7/1(delay_line_in)
  one_tab_4/2(result_out) -> one_tab_7/2(result_in)
  one_tab_4/3(reset_out) -> one_tab_7/3(reset_in)
  one_tab_4/4(enable_out) -> one_tab_7/4(enable_in)

== system sim_model/channelizer/poly_phase_filter1/filter_pipeline_89_taps1/8_taps6 ==
  delay_line_in : Inport
  result_in : Inport  Port=2
  reset_in : Inport  Port=3
  enable_in : Inport  Port=4
  one_tab_1 : Subsystem  mask{impulse_response_matrix=impulse_response_matrix(2,:), N_sub=N_sub}
      mask prompts: impulse_response_matrix "Tab IR"
  one_tab_2 : Subsystem  mask{impulse_response_matrix=impulse_response_matrix(4,:), N_sub=N_sub}
      mask prompts: impulse_response_matrix "Tab IR"
  one_tab_3 : Subsystem  mask{impulse_response_matrix=impulse_response_matrix(3,:), N_sub=N_sub}
      mask prompts: impulse_response_matrix "Tab IR"
  one_tab_4 : Subsystem  mask{impulse_response_matrix=impulse_response_matrix(6,:), N_sub=N_sub}
      mask prompts: impulse_response_matrix "Tab IR"
  one_tab_5 : Subsystem  mask{impulse_response_matrix=impulse_response_matrix(5,:), N_sub=N_sub}
      mask prompts: impulse_response_matrix "Tab IR"
  one_tab_6 : Subsystem  mask{impulse_response_matrix=impulse_response_matrix(8,:), N_sub=N_sub}
      mask prompts: impulse_response_matrix "Tab IR"
  one_tab_7 : Subsystem  mask{impulse_response_matrix=impulse_response_matrix(7,:), N_sub=N_sub}
      mask prompts: impulse_response_matrix "Tab IR"
  one_tab_8 : Subsystem  mask{impulse_response_matrix=impulse_response_matrix(1,:), N_sub=N_sub}
      mask prompts: impulse_response_matrix "Tab IR"
  delay_line_out : Outport
  result_out : Outport  Port=2
  reset_out : Outport  Port=3
  enable_out : Outport  Port=4
  wires:
  one_tab_6/1(delay_line_out) -> delay_line_out/1
  one_tab_6/2(result_out) -> result_out/1
  one_tab_6/3(reset_out) -> reset_out/1
  result_in/1 -> one_tab_8/2(result_in)
  delay_line_in/1 -> one_tab_8/1(delay_line_in)
  reset_in/1 -> one_tab_8/3(reset_in)
  enable_in/1 -> one_tab_8/4(enable_in)
  one_tab_6/4(enable_out) -> enable_out/1
  one_tab_8/1(delay_line_out) -> one_tab_1/1(delay_line_in)
  one_tab_8/2(result_out) -> one_tab_1/2(result_in)
  one_tab_8/3(reset_out) -> one_tab_1/3(reset_in)
  one_tab_8/4(enable_out) -> one_tab_1/4(enable_in)
  one_tab_3/1(delay_line_out) -> one_tab_2/1(delay_line_in)
  one_tab_3/2(result_out) -> one_tab_2/2(result_in)
  one_tab_3/3(reset_out) -> one_tab_2/3(reset_in)
  one_tab_3/4(enable_out) -> one_tab_2/4(enable_in)
  one_tab_1/1(delay_line_out) -> one_tab_3/1(delay_line_in)
  one_tab_1/2(result_out) -> one_tab_3/2(result_in)
  one_tab_1/3(reset_out) -> one_tab_3/3(reset_in)
  one_tab_1/4(enable_out) -> one_tab_3/4(enable_in)
  one_tab_5/1(delay_line_out) -> one_tab_4/1(delay_line_in)
  one_tab_5/2(result_out) -> one_tab_4/2(result_in)
  one_tab_5/3(reset_out) -> one_tab_4/3(reset_in)
  one_tab_5/4(enable_out) -> one_tab_4/4(enable_in)
  one_tab_2/1(delay_line_out) -> one_tab_5/1(delay_line_in)
  one_tab_2/2(result_out) -> one_tab_5/2(result_in)
  one_tab_2/3(reset_out) -> one_tab_5/3(reset_in)
  one_tab_2/4(enable_out) -> one_tab_5/4(enable_in)
  one_tab_7/1(delay_line_out) -> one_tab_6/1(delay_line_in)
  one_tab_7/2(result_out) -> one_tab_6/2(result_in)
  one_tab_7/3(reset_out) -> one_tab_6/3(reset_in)
  one_tab_7/4(enable_out) -> one_tab_6/4(enable_in)
  one_tab_4/1(delay_line_out) -> one_tab_7/1(delay_line_in)
  one_tab_4/2(result_out) -> one_tab_7/2(result_in)
  one_tab_4/3(reset_out) -> one_tab_7/3(reset_in)
  one_tab_4/4(enable_out) -> one_tab_7/4(enable_in)

== system sim_model/channelizer/poly_phase_filter1/filter_pipeline_89_taps1/8_taps7 ==
  delay_line_in : Inport
  result_in : Inport  Port=2
  reset_in : Inport  Port=3
  enable_in : Inport  Port=4
  one_tab_1 : Subsystem  mask{impulse_response_matrix=impulse_response_matrix(2,:), N_sub=N_sub}
      mask prompts: impulse_response_matrix "Tab IR"
  one_tab_2 : Subsystem  mask{impulse_response_matrix=impulse_response_matrix(4,:), N_sub=N_sub}
      mask prompts: impulse_response_matrix "Tab IR"
  one_tab_3 : Subsystem  mask{impulse_response_matrix=impulse_response_matrix(3,:), N_sub=N_sub}
      mask prompts: impulse_response_matrix "Tab IR"
  one_tab_4 : Subsystem  mask{impulse_response_matrix=impulse_response_matrix(6,:), N_sub=N_sub}
      mask prompts: impulse_response_matrix "Tab IR"
  one_tab_5 : Subsystem  mask{impulse_response_matrix=impulse_response_matrix(5,:), N_sub=N_sub}
      mask prompts: impulse_response_matrix "Tab IR"
  one_tab_6 : Subsystem  mask{impulse_response_matrix=impulse_response_matrix(8,:), N_sub=N_sub}
      mask prompts: impulse_response_matrix "Tab IR"
  one_tab_7 : Subsystem  mask{impulse_response_matrix=impulse_response_matrix(7,:), N_sub=N_sub}
      mask prompts: impulse_response_matrix "Tab IR"
  one_tab_8 : Subsystem  mask{impulse_response_matrix=impulse_response_matrix(1,:), N_sub=N_sub}
      mask prompts: impulse_response_matrix "Tab IR"
  delay_line_out : Outport
  result_out : Outport  Port=2
  reset_out : Outport  Port=3
  enable_out : Outport  Port=4
  wires:
  one_tab_6/1(delay_line_out) -> delay_line_out/1
  one_tab_6/2(result_out) -> result_out/1
  one_tab_6/3(reset_out) -> reset_out/1
  result_in/1 -> one_tab_8/2(result_in)
  delay_line_in/1 -> one_tab_8/1(delay_line_in)
  reset_in/1 -> one_tab_8/3(reset_in)
  enable_in/1 -> one_tab_8/4(enable_in)
  one_tab_6/4(enable_out) -> enable_out/1
  one_tab_8/1(delay_line_out) -> one_tab_1/1(delay_line_in)
  one_tab_8/2(result_out) -> one_tab_1/2(result_in)
  one_tab_8/3(reset_out) -> one_tab_1/3(reset_in)
  one_tab_8/4(enable_out) -> one_tab_1/4(enable_in)
  one_tab_3/1(delay_line_out) -> one_tab_2/1(delay_line_in)
  one_tab_3/2(result_out) -> one_tab_2/2(result_in)
  one_tab_3/3(reset_out) -> one_tab_2/3(reset_in)
  one_tab_3/4(enable_out) -> one_tab_2/4(enable_in)
  one_tab_1/1(delay_line_out) -> one_tab_3/1(delay_line_in)
  one_tab_1/2(result_out) -> one_tab_3/2(result_in)
  one_tab_1/3(reset_out) -> one_tab_3/3(reset_in)
  one_tab_1/4(enable_out) -> one_tab_3/4(enable_in)
  one_tab_5/1(delay_line_out) -> one_tab_4/1(delay_line_in)
  one_tab_5/2(result_out) -> one_tab_4/2(result_in)
  one_tab_5/3(reset_out) -> one_tab_4/3(reset_in)
  one_tab_5/4(enable_out) -> one_tab_4/4(enable_in)
  one_tab_2/1(delay_line_out) -> one_tab_5/1(delay_line_in)
  one_tab_2/2(result_out) -> one_tab_5/2(result_in)
  one_tab_2/3(reset_out) -> one_tab_5/3(reset_in)
  one_tab_2/4(enable_out) -> one_tab_5/4(enable_in)
  one_tab_7/1(delay_line_out) -> one_tab_6/1(delay_line_in)
  one_tab_7/2(result_out) -> one_tab_6/2(result_in)
  one_tab_7/3(reset_out) -> one_tab_6/3(reset_in)
  one_tab_7/4(enable_out) -> one_tab_6/4(enable_in)
  one_tab_4/1(delay_line_out) -> one_tab_7/1(delay_line_in)
  one_tab_4/2(result_out) -> one_tab_7/2(result_in)
  one_tab_4/3(reset_out) -> one_tab_7/3(reset_in)
  one_tab_4/4(enable_out) -> one_tab_7/4(enable_in)

== system sim_model/channelizer/poly_phase_filter1/filter_pipeline_89_taps1/8_taps8 ==
  delay_line_in : Inport
  result_in : Inport  Port=2
  reset_in : Inport  Port=3
  enable_in : Inport  Port=4
  one_tab_1 : Subsystem  mask{impulse_response_matrix=impulse_response_matrix(2,:), N_sub=N_sub}
      mask prompts: impulse_response_matrix "Tab IR"
  one_tab_2 : Subsystem  mask{impulse_response_matrix=impulse_response_matrix(4,:), N_sub=N_sub}
      mask prompts: impulse_response_matrix "Tab IR"
  one_tab_3 : Subsystem  mask{impulse_response_matrix=impulse_response_matrix(3,:), N_sub=N_sub}
      mask prompts: impulse_response_matrix "Tab IR"
  one_tab_4 : Subsystem  mask{impulse_response_matrix=impulse_response_matrix(6,:), N_sub=N_sub}
      mask prompts: impulse_response_matrix "Tab IR"
  one_tab_5 : Subsystem  mask{impulse_response_matrix=impulse_response_matrix(5,:), N_sub=N_sub}
      mask prompts: impulse_response_matrix "Tab IR"
  one_tab_6 : Subsystem  mask{impulse_response_matrix=impulse_response_matrix(8,:), N_sub=N_sub}
      mask prompts: impulse_response_matrix "Tab IR"
  one_tab_7 : Subsystem  mask{impulse_response_matrix=impulse_response_matrix(7,:), N_sub=N_sub}
      mask prompts: impulse_response_matrix "Tab IR"
  one_tab_8 : Subsystem  mask{impulse_response_matrix=impulse_response_matrix(1,:), N_sub=N_sub}
      mask prompts: impulse_response_matrix "Tab IR"
  delay_line_out : Outport
  result_out : Outport  Port=2
  reset_out : Outport  Port=3
  enable_out : Outport  Port=4
  wires:
  one_tab_6/1(delay_line_out) -> delay_line_out/1
  one_tab_6/2(result_out) -> result_out/1
  one_tab_6/3(reset_out) -> reset_out/1
  result_in/1 -> one_tab_8/2(result_in)
  delay_line_in/1 -> one_tab_8/1(delay_line_in)
  reset_in/1 -> one_tab_8/3(reset_in)
  enable_in/1 -> one_tab_8/4(enable_in)
  one_tab_6/4(enable_out) -> enable_out/1
  one_tab_8/1(delay_line_out) -> one_tab_1/1(delay_line_in)
  one_tab_8/2(result_out) -> one_tab_1/2(result_in)
  one_tab_8/3(reset_out) -> one_tab_1/3(reset_in)
  one_tab_8/4(enable_out) -> one_tab_1/4(enable_in)
  one_tab_3/1(delay_line_out) -> one_tab_2/1(delay_line_in)
  one_tab_3/2(result_out) -> one_tab_2/2(result_in)
  one_tab_3/3(reset_out) -> one_tab_2/3(reset_in)
  one_tab_3/4(enable_out) -> one_tab_2/4(enable_in)
  one_tab_1/1(delay_line_out) -> one_tab_3/1(delay_line_in)
  one_tab_1/2(result_out) -> one_tab_3/2(result_in)
  one_tab_1/3(reset_out) -> one_tab_3/3(reset_in)
  one_tab_1/4(enable_out) -> one_tab_3/4(enable_in)
  one_tab_5/1(delay_line_out) -> one_tab_4/1(delay_line_in)
  one_tab_5/2(result_out) -> one_tab_4/2(result_in)
  one_tab_5/3(reset_out) -> one_tab_4/3(reset_in)
  one_tab_5/4(enable_out) -> one_tab_4/4(enable_in)
  one_tab_2/1(delay_line_out) -> one_tab_5/1(delay_line_in)
  one_tab_2/2(result_out) -> one_tab_5/2(result_in)
  one_tab_2/3(reset_out) -> one_tab_5/3(reset_in)
  one_tab_2/4(enable_out) -> one_tab_5/4(enable_in)
  one_tab_7/1(delay_line_out) -> one_tab_6/1(delay_line_in)
  one_tab_7/2(result_out) -> one_tab_6/2(result_in)
  one_tab_7/3(reset_out) -> one_tab_6/3(reset_in)
  one_tab_7/4(enable_out) -> one_tab_6/4(enable_in)
  one_tab_4/1(delay_line_out) -> one_tab_7/1(delay_line_in)
  one_tab_4/2(result_out) -> one_tab_7/2(result_in)
  one_tab_4/3(reset_out) -> one_tab_7/3(reset_in)
  one_tab_4/4(enable_out) -> one_tab_7/4(enable_in)

== system sim_model/channelizer/poly_phase_filter1/filter_pipeline_89_taps1/8_taps9 ==
  delay_line_in : Inport
  result_in : Inport  Port=2
  reset_in : Inport  Port=3
  enable_in : Inport  Port=4
  one_tab_1 : Subsystem  mask{impulse_response_matrix=impulse_response_matrix(2,:), N_sub=N_sub}
      mask prompts: impulse_response_matrix "Tab IR"
  one_tab_2 : Subsystem  mask{impulse_response_matrix=impulse_response_matrix(4,:), N_sub=N_sub}
      mask prompts: impulse_response_matrix "Tab IR"
  one_tab_3 : Subsystem  mask{impulse_response_matrix=impulse_response_matrix(3,:), N_sub=N_sub}
      mask prompts: impulse_response_matrix "Tab IR"
  one_tab_4 : Subsystem  mask{impulse_response_matrix=impulse_response_matrix(6,:), N_sub=N_sub}
      mask prompts: impulse_response_matrix "Tab IR"
  one_tab_5 : Subsystem  mask{impulse_response_matrix=impulse_response_matrix(5,:), N_sub=N_sub}
      mask prompts: impulse_response_matrix "Tab IR"
  one_tab_6 : Subsystem  mask{impulse_response_matrix=impulse_response_matrix(8,:), N_sub=N_sub}
      mask prompts: impulse_response_matrix "Tab IR"
  one_tab_7 : Subsystem  mask{impulse_response_matrix=impulse_response_matrix(7,:), N_sub=N_sub}
      mask prompts: impulse_response_matrix "Tab IR"
  one_tab_8 : Subsystem  mask{impulse_response_matrix=impulse_response_matrix(1,:), N_sub=N_sub}
      mask prompts: impulse_response_matrix "Tab IR"
  delay_line_out : Outport
  result_out : Outport  Port=2
  reset_out : Outport  Port=3
  enable_out : Outport  Port=4
  wires:
  one_tab_6/1(delay_line_out) -> delay_line_out/1
  one_tab_6/2(result_out) -> result_out/1
  one_tab_6/3(reset_out) -> reset_out/1
  result_in/1 -> one_tab_8/2(result_in)
  delay_line_in/1 -> one_tab_8/1(delay_line_in)
  reset_in/1 -> one_tab_8/3(reset_in)
  enable_in/1 -> one_tab_8/4(enable_in)
  one_tab_6/4(enable_out) -> enable_out/1
  one_tab_8/1(delay_line_out) -> one_tab_1/1(delay_line_in)
  one_tab_8/2(result_out) -> one_tab_1/2(result_in)
  one_tab_8/3(reset_out) -> one_tab_1/3(reset_in)
  one_tab_8/4(enable_out) -> one_tab_1/4(enable_in)
  one_tab_3/1(delay_line_out) -> one_tab_2/1(delay_line_in)
  one_tab_3/2(result_out) -> one_tab_2/2(result_in)
  one_tab_3/3(reset_out) -> one_tab_2/3(reset_in)
  one_tab_3/4(enable_out) -> one_tab_2/4(enable_in)
  one_tab_1/1(delay_line_out) -> one_tab_3/1(delay_line_in)
  one_tab_1/2(result_out) -> one_tab_3/2(result_in)
  one_tab_1/3(reset_out) -> one_tab_3/3(reset_in)
  one_tab_1/4(enable_out) -> one_tab_3/4(enable_in)
  one_tab_5/1(delay_line_out) -> one_tab_4/1(delay_line_in)
  one_tab_5/2(result_out) -> one_tab_4/2(result_in)
  one_tab_5/3(reset_out) -> one_tab_4/3(reset_in)
  one_tab_5/4(enable_out) -> one_tab_4/4(enable_in)
  one_tab_2/1(delay_line_out) -> one_tab_5/1(delay_line_in)
  one_tab_2/2(result_out) -> one_tab_5/2(result_in)
  one_tab_2/3(reset_out) -> one_tab_5/3(reset_in)
  one_tab_2/4(enable_out) -> one_tab_5/4(enable_in)
  one_tab_7/1(delay_line_out) -> one_tab_6/1(delay_line_in)
  one_tab_7/2(result_out) -> one_tab_6/2(result_in)
  one_tab_7/3(reset_out) -> one_tab_6/3(reset_in)
  one_tab_7/4(enable_out) -> one_tab_6/4(enable_in)
  one_tab_4/1(delay_line_out) -> one_tab_7/1(delay_line_in)
  one_tab_4/2(result_out) -> one_tab_7/2(result_in)
  one_tab_4/3(reset_out) -> one_tab_7/3(reset_in)
  one_tab_4/4(enable_out) -> one_tab_7/4(enable_in)
